simulink model "equilibrium_points"  (R2022b)
settings: Solver=ode113  StartTime=-5  StopTime=5  MaxStep=4.0  RelTol=1e-3
settings Model: Creator=anver  LastModifiedBy=anver
settings SolverCC: ZeroCrossAlgorithm=Adaptive

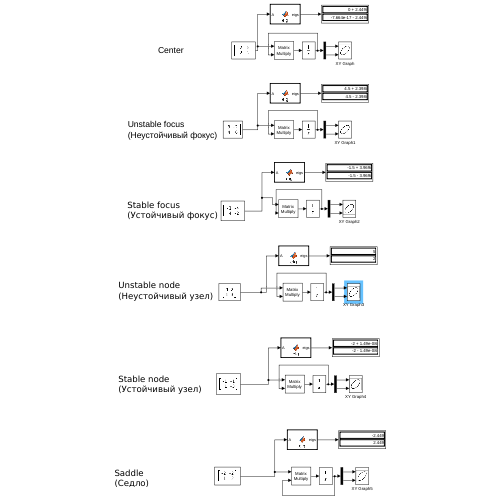
[thumbnail: Simulink's stored preview of the top-level diagram]
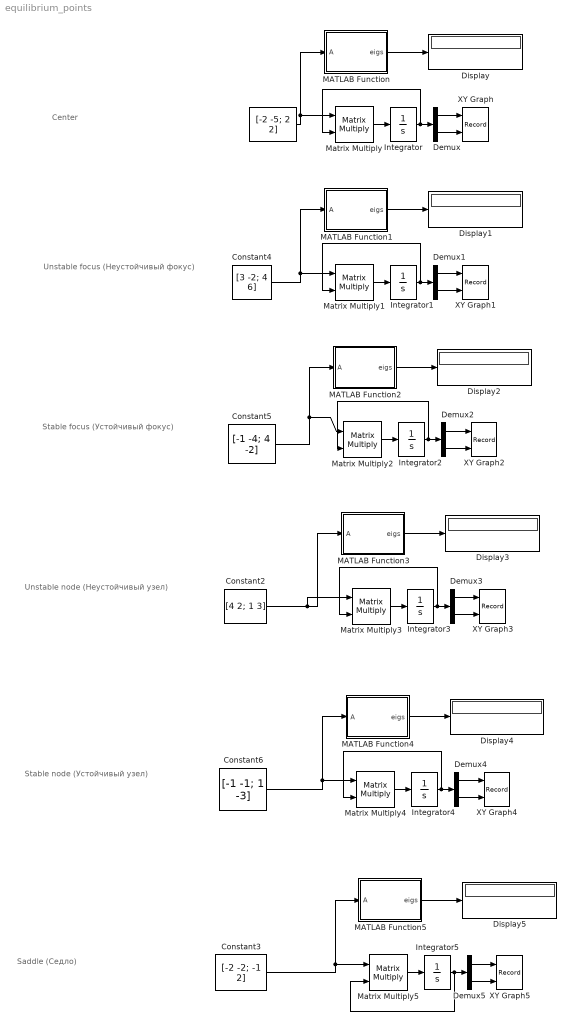
== system equilibrium_points ==
  note: Saddle
      | (Седло)
  note: Stable node
      | (Устойчивый узел)
  note: Unstable node
      | (Неустойчивый узел)
  note: Stable focus
      | (Устойчивый фокус)
  note: Unstable focus
      | (Неустойчивый фокус)
  note: Center
  " " : Constant  Value=[-2 -5; 2 2]  VectorParams1D=off
  Constant2 : Constant  Value=[4 2; 1 3]
  Constant3 : Constant  Value=[-2 -2; -1 2]
  Constant4 : Constant  Value=[3 -2; 4 6]
  Constant5 : Constant  Value=[-1 -4; 4 -2]
  Constant6 : Constant  Value=[-1 -1; 1 -3]
  Demux{,1..5} (6 alike) : Demux  Outputs=2
  Display{,1..5} (6 alike) : Display
  Integrator : Integrator  InitialCondition=[1; 1]
  Integrator1 : Integrator  InitialCondition=[1; 1]
  Integrator2 : Integrator  InitialCondition=[1, 1]
  Integrator3 : Integrator  InitialCondition=[1, 1]
  Integrator4 : Integrator  InitialCondition=[1 -1]
  Integrator5 : Integrator  InitialCondition=[1, 1]
  MATLAB Function : MATLAB Function  TreatAsAtomicUnit=on
  MATLAB Function1 : MATLAB Function  TreatAsAtomicUnit=on
  MATLAB Function2 : MATLAB Function  TreatAsAtomicUnit=on
  MATLAB Function3 : MATLAB Function  TreatAsAtomicUnit=on
  MATLAB Function4 : MATLAB Function  TreatAsAtomicUnit=on
  MATLAB Function5 : MATLAB Function  TreatAsAtomicUnit=on
  Matrix Multiply{,1..5} (6 alike) : Product  Multiplication=Matrix(*)
  XY Graph : Record  FileSettingsInternal="{\"entries\":[{\"content\":{\"excelSettings\":{\"content\":{},\"type\":\"Streamout.ExcelSettings\"}},\"type\":\"Streamout.FileSettingStorage\",\"uuid\":\"5ba9cb58-1892-4736-b0fb-b51552328347\"}],\"packageUris\":[\"http://schema.mathworks.com/mf0/streamout_blocks/R2020a\"],\"version\":\"1.0\"}"  Layout=[1 1]  SignalsInternal="{\"entries\":[{\"content\":{\"signals\":[{\"content\":{\"blockPath\":[\"equilibrium_points/XY Graph\"],\"channel\":[],\"dimensions\":[1],\"domain\":\"equilibrium_points/XY Graph\",\"lineColor\":\"#a2142f\",\"plots\":[1],\"port\":1,\"sid\":[\"\"],\"signalID\":996,\"signalName\":\"Demux:1\"},\"type\":\"RecordBlkView.Signal\",\"uuid\":\"8ee31b2e-c810-4496-bf45-e3850a45951f\"},{\"content\":{\"blockPath\":[\"equilibrium_points/XY Graph\"],\"channel\":[],\"dimensions\":[1],\"domain\":\"equilibrium_points/XY Graph\",\"lineColor\":\"#139fff\",\"plots\":[1],\"port\":2,\"sid\":[\"\"],\"signalID\":1000,\"signalName\":\"Demux:2\"},\"type\":\"RecordBlkView.Signal\",\"uuid\":\"7ca83951-d0e9-4205-8030-7fbe9e126d03\"}]},\"type\":\"RecordBlkView.InputSignals\",\"uuid\":\"f964ffeb-f08f-465e-9261-1e37639215ae\"}],\"packageUris\":[\"http://schema.mathworks.com/mf0/streamout_blocks/R2020a\"],\"version\":\"1.0\"}"  VisualizationBindings="{\"xyplotplugin\":{\"info\":[{\"series\":[{\"bindingParametersList\":[{\"parameter\":\"X-Axis\",\"signalID\":996,\"signalName\":\"Demux:1\"},{\"parameter\":\"Y-Axis\",\"signalID\":1000,\"signalName\":\"Demux:2\"}],\"seriesID\":56605}],\"subplotID\":1}]}}"  CompatibilityTag=XY  st=-1
  XY Graph1 : Record  FileSettingsInternal="{\"entries\":[{\"content\":{\"excelSettings\":{\"content\":{},\"type\":\"Streamout.ExcelSettings\"}},\"type\":\"Streamout.FileSettingStorage\",\"uuid\":\"90a31ab9-f841-460b-a2f2-54c253a22699\"}],\"packageUris\":[\"http://schema.mathworks.com/mf0/streamout_blocks/R2020a\"],\"version\":\"1.0\"}"  Layout=[1 1]  SignalsInternal="{\"entries\":[{\"content\":{\"signals\":[{\"content\":{\"blockPath\":[\"equilibrium_points/XY Graph1\"],\"channel\":[],\"dimensions\":[1],\"domain\":\"equilibrium_points/XY Graph1\",\"lineColor\":\"#a2142f\",\"plots\":[1],\"port\":1,\"sid\":[\"\"],\"signalID\":1020,\"signalName\":\"Demux1:1\"},\"type\":\"RecordBlkView.Signal\",\"uuid\":\"16337b76-6d05-4d02-9ca3-4e0a2bc79a4e\"},{\"content\":{\"blockPath\":[\"equilibrium_points/XY Graph1\"],\"channel\":[],\"dimensions\":[1],\"domain\":\"equilibrium_points/XY Graph1\",\"lineColor\":\"#139fff\",\"plots\":[1],\"port\":2,\"sid\":[\"\"],\"signalID\":1024,\"signalName\":\"Demux1:2\"},\"type\":\"RecordBlkView.Signal\",\"uuid\":\"2185b3fc-28ad-469e-bc31-6f4de757a18d\"}]},\"type\":\"RecordBlkView.InputSignals\",\"uuid\":\"18fb4397-b3cc-410d-bdf1-d16aca643980\"}],\"packageUris\":[\"http://schema.mathworks.com/mf0/streamout_blocks/R2020a\"],\"version\":\"1.0\"}"  VisualizationBindings="{\"xyplotplugin\":{\"info\":[{\"series\":[{\"bindingParametersList\":[{\"parameter\":\"X-Axis\",\"signalID\":1020,\"signalName\":\"Demux1:1\"},{\"parameter\":\"Y-Axis\",\"signalID\":1024,\"signalName\":\"Demux1:2\"}],\"seriesID\":17990}],\"subplotID\":1}]}}"  CompatibilityTag=XY  st=-1
  XY Graph2 : Record  FileSettingsInternal="{\"entries\":[{\"content\":{\"excelSettings\":{\"content\":{},\"type\":\"Streamout.ExcelSettings\"}},\"type\":\"Streamout.FileSettingStorage\",\"uuid\":\"b670f568-656d-4987-b8c3-0f73c2f253b8\"}],\"packageUris\":[\"http://schema.mathworks.com/mf0/streamout_blocks/R2020a\"],\"version\":\"1.0\"}"  Layout=[1 1]  SignalsInternal="{\"entries\":[{\"content\":{\"signals\":[{\"content\":{\"blockPath\":[\"equilibrium_points/XY Graph2\"],\"channel\":[],\"dimensions\":[1],\"domain\":\"equilibrium_points/XY Graph2\",\"lineColor\":\"#a2142f\",\"plots\":[1],\"port\":1,\"sid\":[\"\"],\"signalID\":1028,\"signalName\":\"Demux2:1\"},\"type\":\"RecordBlkView.Signal\",\"uuid\":\"3d2b5602-d316-4ec7-acfc-86114c820535\"},{\"content\":{\"blockPath\":[\"equilibrium_points/XY Graph2\"],\"channel\":[],\"dimensions\":[1],\"domain\":\"equilibrium_points/XY Graph2\",\"lineColor\":\"#139fff\",\"plots\":[1],\"port\":2,\"sid\":[\"\"],\"signalID\":1032,\"signalName\":\"Demux2:2\"},\"type\":\"RecordBlkView.Signal\",\"uuid\":\"88e7b222-2427-45e2-a93e-30f7102c3b82\"}]},\"type\":\"RecordBlkView.InputSignals\",\"uuid\":\"bf206ba8-bcdf-4768-8ddf-5e07e1d1c2c1\"}],\"packageUris\":[\"http://schema.mathworks.com/mf0/streamout_blocks/R2020a\"],\"version\":\"1.0\"}"  VisualizationBindings="{\"xyplotplugin\":{\"info\":[{\"series\":[{\"bindingParametersList\":[{\"parameter\":\"X-Axis\",\"signalID\":1028,\"signalName\":\"Demux2:1\"},{\"parameter\":\"Y-Axis\",\"signalID\":1032,\"signalName\":\"Demux2:2\"}],\"seriesID\":26207}],\"subplotID\":1}]}}"  CompatibilityTag=XY  st=-1
  XY Graph3 : Record  FileSettingsInternal="{\"entries\":[{\"content\":{\"excelSettings\":{\"content\":{},\"type\":\"Streamout.ExcelSettings\"}},\"type\":\"Streamout.FileSettingStorage\",\"uuid\":\"576b0026-31d3-4fbd-9a62-7a169cad687e\"}],\"packageUris\":[\"http://schema.mathworks.com/mf0/streamout_blocks/R2020a\"],\"version\":\"1.0\"}"  Layout=[1 1]  SignalsInternal="{\"entries\":[{\"content\":{\"signals\":[{\"content\":{\"blockPath\":[\"equilibrium_points/XY Graph3\"],\"channel\":[],\"dimensions\":[1],\"domain\":\"equilibrium_points/XY Graph3\",\"lineColor\":\"#a2142f\",\"plots\":[1],\"port\":1,\"sid\":[\"\"],\"signalID\":1004,\"signalName\":\"Demux3:1\"},\"type\":\"RecordBlkView.Signal\",\"uuid\":\"5c71d26b-1578-49ec-a98c-d994a0e6477b\"},{\"content\":{\"blockPath\":[\"equilibrium_points/XY Graph3\"],\"channel\":[],\"dimensions\":[1],\"domain\":\"equilibrium_points/XY Graph3\",\"lineColor\":\"#139fff\",\"plots\":[1],\"port\":2,\"sid\":[\"\"],\"signalID\":1008,\"signalName\":\"Demux3:2\"},\"type\":\"RecordBlkView.Signal\",\"uuid\":\"a8c2bb67-cf90-427d-8745-3a0bacc8e481\"}]},\"type\":\"RecordBlkView.InputSignals\",\"uuid\":\"ca1ecf62-eab6-4967-af64-db16bee20c1a\"}],\"packageUris\":[\"http://schema.mathworks.com/mf0/streamout_blocks/R2020a\"],\"version\":\"1.0\"}"  VisualizationBindings="{\"xyplotplugin\":{\"info\":[{\"series\":[{\"bindingParametersList\":[{\"parameter\":\"X-Axis\",\"signalID\":1004,\"signalName\":\"Demux3:1\"},{\"parameter\":\"Y-Axis\",\"signalID\":1008,\"signalName\":\"Demux3:2\"}],\"seriesID\":36648}],\"subplotID\":1}]}}"  CompatibilityTag=XY  st=-1
  XY Graph4 : Record  FileSettingsInternal="{\"entries\":[{\"content\":{\"excelSettings\":{\"content\":{},\"type\":\"Streamout.ExcelSettings\"}},\"type\":\"Streamout.FileSettingStorage\",\"uuid\":\"65c71d67-6847-4a46-9140-01ecd77b0d4b\"}],\"packageUris\":[\"http://schema.mathworks.com/mf0/streamout_blocks/R2020a\"],\"version\":\"1.0\"}"  Layout=[1 1]  SignalsInternal="{\"entries\":[{\"content\":{\"signals\":[{\"content\":{\"blockPath\":[\"equilibrium_points/XY Graph4\"],\"channel\":[],\"dimensions\":[1],\"domain\":\"equilibrium_points/XY Graph4\",\"lineColor\":\"#a2142f\",\"plots\":[1],\"port\":1,\"sid\":[\"\"],\"signalID\":1036,\"signalName\":\"Demux4:1\"},\"type\":\"RecordBlkView.Signal\",\"uuid\":\"4b295772-ca43-4c82-8759-12492f1ba9fc\"},{\"content\":{\"blockPath\":[\"equilibrium_points/XY Graph4\"],\"channel\":[],\"dimensions\":[1],\"domain\":\"equilibrium_points/XY Graph4\",\"lineColor\":\"#139fff\",\"plots\":[1],\"port\":2,\"sid\":[\"\"],\"signalID\":1040,\"signalName\":\"Demux4:2\"},\"type\":\"RecordBlkView.Signal\",\"uuid\":\"2e9a5f0f-86f5-4847-ab06-fc978e03dda3\"}]},\"type\":\"RecordBlkView.InputSignals\",\"uuid\":\"764788e9-d75a-4fdc-88e8-13140d855fda\"}],\"packageUris\":[\"http://schema.mathworks.com/mf0/streamout_blocks/R2020a\"],\"version\":\"1.0\"}"  VisualizationBindings="{\"xyplotplugin\":{\"info\":[{\"series\":[{\"bindingParametersList\":[{\"parameter\":\"X-Axis\",\"signalID\":1036,\"signalName\":\"Demux4:1\"},{\"parameter\":\"Y-Axis\",\"signalID\":1040,\"signalName\":\"Demux4:2\"}],\"seriesID\":25257}],\"subplotID\":1}]}}"  CompatibilityTag=XY  st=-1
  XY Graph5 : Record  FileSettingsInternal="{\"entries\":[{\"content\":{\"excelSettings\":{\"content\":{},\"type\":\"Streamout.ExcelSettings\"}},\"type\":\"Streamout.FileSettingStorage\",\"uuid\":\"b8045a63-21fc-4349-8645-e5cc530c865c\"}],\"packageUris\":[\"http://schema.mathworks.com/mf0/streamout_blocks/R2020a\"],\"version\":\"1.0\"}"  Layout=[1 1]  SignalsInternal="{\"entries\":[{\"content\":{\"signals\":[{\"content\":{\"blockPath\":[\"equilibrium_points/XY Graph5\"],\"channel\":[],\"dimensions\":[1],\"domain\":\"equilibrium_points/XY Graph5\",\"lineColor\":\"#a2142f\",\"plots\":[1],\"port\":1,\"sid\":[\"\"],\"signalID\":1012,\"signalName\":\"Demux5:1\"},\"type\":\"RecordBlkView.Signal\",\"uuid\":\"8bb5e75a-ba78-45e6-9c56-6941ec562ad6\"},{\"content\":{\"blockPath\":[\"equilibrium_points/XY Graph5\"],\"channel\":[],\"dimensions\":[1],\"domain\":\"equilibrium_points/XY Graph5\",\"lineColor\":\"#139fff\",\"plots\":[1],\"port\":2,\"sid\":[\"\"],\"signalID\":1016,\"signalName\":\"Demux5:2\"},\"type\":\"RecordBlkView.Signal\",\"uuid\":\"1cc1c057-19e4-4cc8-94a5-65827af7e705\"}]},\"type\":\"RecordBlkView.InputSignals\",\"uuid\":\"28cf081a-5777-4b39-af01-63441b329d7a\"}],\"packageUris\":[\"http://schema.mathworks.com/mf0/streamout_blocks/R2020a\"],\"version\":\"1.0\"}"  VisualizationBindings="{\"xyplotplugin\":{\"info\":[{\"series\":[{\"bindingParametersList\":[{\"parameter\":\"X-Axis\",\"signalID\":1012,\"signalName\":\"Demux5:1\"},{\"parameter\":\"Y-Axis\",\"signalID\":1016,\"signalName\":\"Demux5:2\"}],\"seriesID\":34210}],\"subplotID\":1}]}}"  CompatibilityTag=XY  st=-1
  wires:
  Matrix Multiply/1 -> Integrator/1
  Integrator/1 -> Matrix Multiply/2, Demux/1
  Demux/1 -> XY Graph/1
  Demux/2 -> XY Graph/2
  MATLAB Function/1(eigs) -> Display/1
  MATLAB Function1/1(eigs) -> Display1/1
  Demux1/1 -> XY Graph1/1
  Demux1/2 -> XY Graph1/2
  Constant4/1 -> Matrix Multiply1/1, MATLAB Function1/1(A)
  Matrix Multiply1/1 -> Integrator1/1
  Integrator1/1 -> Matrix Multiply1/2, Demux1/1
  Integrator2/1 -> Matrix Multiply2/2, Demux2/1
  Constant5/1 -> Matrix Multiply2/1, MATLAB Function2/1(A)
  Matrix Multiply2/1 -> Integrator2/1
  MATLAB Function2/1(eigs) -> Display2/1
  Demux2/1 -> XY Graph2/1
  Demux2/2 -> XY Graph2/2
  Integrator3/1 -> Matrix Multiply3/2, Demux3/1
  Constant2/1 -> Matrix Multiply3/1, MATLAB Function3/1(A)
  MATLAB Function3/1(eigs) -> Display3/1
  Matrix Multiply3/1 -> Integrator3/1
  Demux3/1 -> XY Graph3/1
  Demux3/2 -> XY Graph3/2
  Demux4/2 -> XY Graph4/2
  Constant6/1 -> MATLAB Function4/1(A), Matrix Multiply4/1
  Integrator4/1 -> Matrix Multiply4/2, Demux4/1
  Matrix Multiply4/1 -> Integrator4/1
  MATLAB Function4/1(eigs) -> Display4/1
  Demux4/1 -> XY Graph4/1
  Matrix Multiply5/1 -> Integrator5/1
  Constant3/1 -> MATLAB Function5/1(A), Matrix Multiply5/1
  Demux5/2 -> XY Graph5/2
  MATLAB Function5/1(eigs) -> Display5/1
  Demux5/1 -> XY Graph5/1
  " "/1 -> MATLAB Function/1(A), Matrix Multiply/1
  Integrator5/1 -> Matrix Multiply5/2, Demux5/1

== matlab function equilibrium_points/MATLAB Function ==
  data: A input; eigs output
function eigs = eig(A)

eigs = eig(A);

== matlab function equilibrium_points/MATLAB Function2 ==
  data: A input; eigs output
function eigs = eig(A)

eigs = eig(A);

== matlab function equilibrium_points/MATLAB Function3 ==
  data: A input; eigs output
function eigs = eig(A)

eigs = eig(A);

== matlab function equilibrium_points/MATLAB Function4 ==
  data: A input; eigs output
function eigs = eig(A)

eigs = eig(A);

== matlab function equilibrium_points/MATLAB Function5 ==
  data: A input; eigs output
function eigs = eig(A)

eigs = eig(A);

== matlab function equilibrium_points/MATLAB Function1 ==
  data: A input; eigs output
function eigs = eig(A)

eigs = eig(A);
